simulink library "lib_Hand"  (R2022b)
settings: Solver=VariableStepAuto  StartTime=0.0  StopTime=10.0  RelTol=1e-3
settings Model: Creator=li_ju  LastModifiedBy=ge26jow

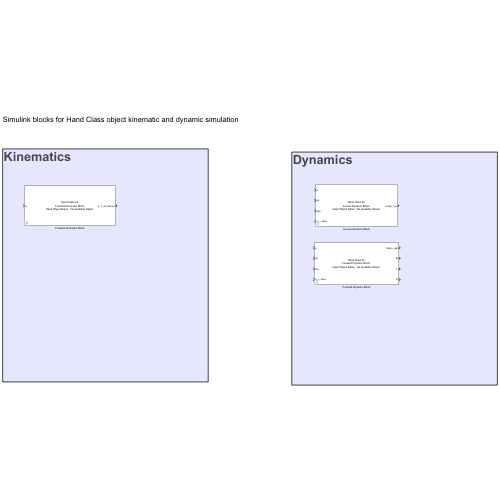
[thumbnail: Simulink's stored preview of the top-level diagram]
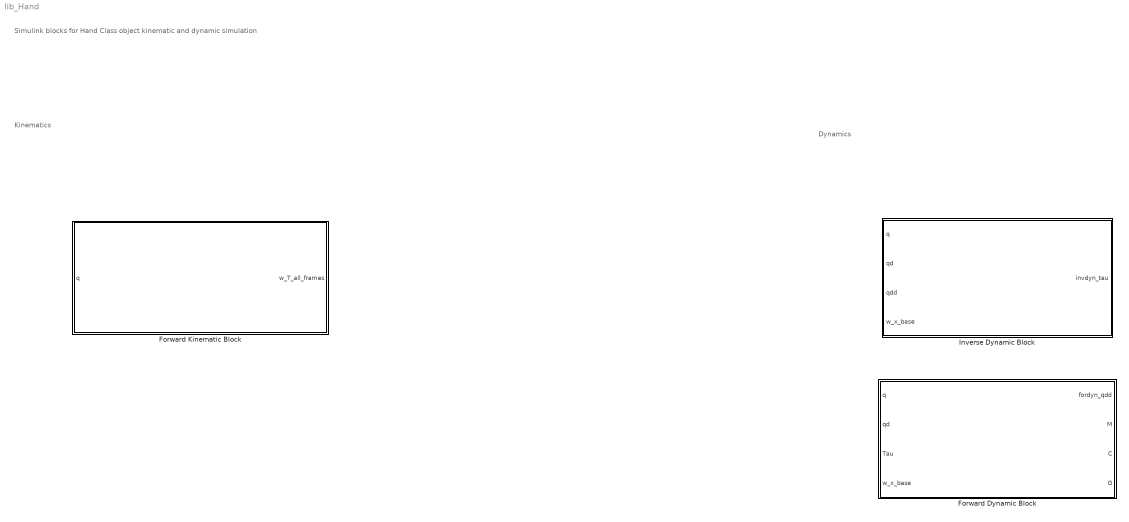
== system lib_Hand ==
  note: Kinematics
  note: Simulink blocks for Hand Class object kinematic and dynamic simulation
  note: Dynamics
  Forward Dynamic Block : Subsystem  mask{hand=0}
      mask prompts: hand "Hand Model Object"
      mask init:
      | if isa(hand,"Hand")
      |        handname = hand.name;
      |    else
      |         handname = 'No Available Object';
      |    end
      mask Display:
      | fprintf(['Hand Class lib \n' ...
      |     'Forward Dynamic Block \n' ...
      |     'Hand Object Name:  %s '], handname)
  Forward Kinematic Block : Subsystem  mask{hand=0}
      mask prompts: hand "Hand Model Object"
      mask init:
      | if isa(hand,"Hand")
      |        handname = hand.name;
      |    else
      |         handname = 'No Available Object';
      |    end
      mask Display:
      | fprintf(['Hand Class lib \n' ...
      |     'Forward Kinematic Block \n' ...
      |     'Hand Object Name:  %s '], handname)
  Inverse Dynamic Block : Subsystem  mask{hand=0}
      mask prompts: hand "Hand Model Object"
      mask init:
      | if isa(hand,"Hand")
      |        handname = hand.name;
      |    else
      |         handname = 'No Available Object';
      |    end
      mask Display:
      | fprintf(['Hand Class lib \n' ...
      |     'Inverse Dynamic Block \n' ...
      |     'Hand Object Name:  %s '], handname)

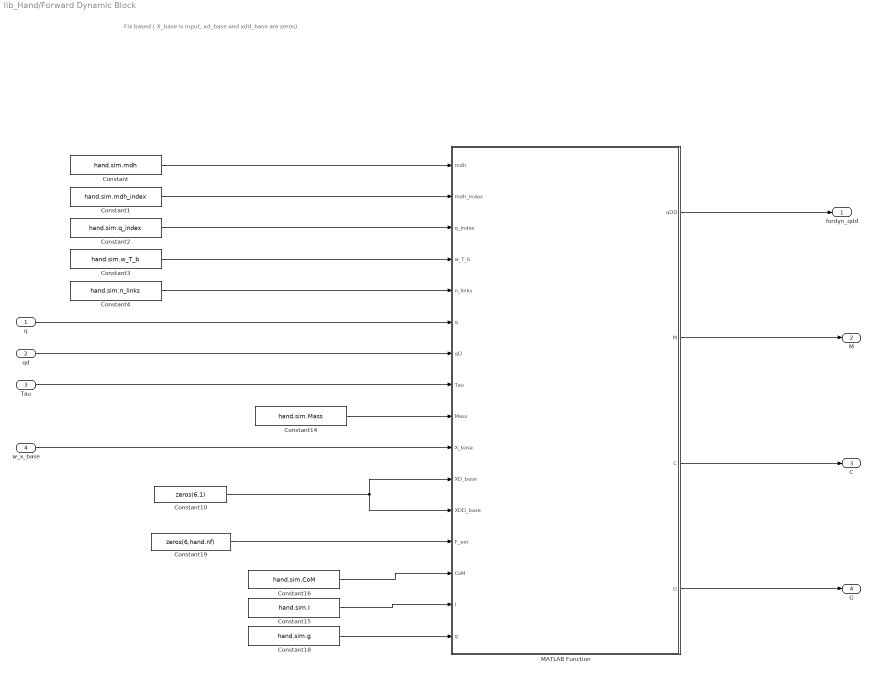
== system lib_Hand/Forward Dynamic Block ==
  note: Fix based ( X_base is input, xd_base and xdd_base are zeros)
  q : Inport
  qd : Inport  Port=2
  Tau : Inport  Port=3
  w_x_base : Inport  Port=4
  Constant : Constant  Value=hand.sim.mdh
  Constant1 : Constant  Value=hand.sim.mdh_index
  Constant10 : Constant  Value=zeros(6,1)  VectorParams1D=off
  Constant14 : Constant  Value=hand.sim.Mass  VectorParams1D=off
  Constant15 : Constant  Value=hand.sim.I
  Constant16 : Constant  Value=hand.sim.CoM
  Constant18 : Constant  Value=hand.sim.g  VectorParams1D=off
  Constant19 : Constant  Value=zeros(6,hand.nf)
  Constant2 : Constant  Value=hand.sim.q_index
  Constant3 : Constant  Value=hand.sim.w_T_b
  Constant4 : Constant  Value=hand.sim.n_links  VectorParams1D=off
  MATLAB Function : MATLAB Function  TreatAsAtomicUnit=on
  fordyn_qdd : Outport
  M : Outport  Port=2
  C : Outport  Port=3
  G : Outport  Port=4
  wires:
  Constant14/1 -> MATLAB Function/9(Mass)
  MATLAB Function/1(qDD) -> fordyn_qdd/1
  Constant10/1 -> MATLAB Function/12(XDD_base), MATLAB Function/11(XD_base)
  Constant15/1 -> MATLAB Function/15(I)
  Constant19/1 -> MATLAB Function/13(F_ext)
  Constant16/1 -> MATLAB Function/14(CoM)
  qd/1 -> MATLAB Function/7(qD)
  Constant2/1 -> MATLAB Function/3(q_index)
  q/1 -> MATLAB Function/6(q)
  Constant/1 -> MATLAB Function/1(mdh)
  Constant3/1 -> MATLAB Function/4(w_T_b)
  Constant1/1 -> MATLAB Function/2(mdh_index)
  Constant18/1 -> MATLAB Function/16(g)
  Constant4/1 -> MATLAB Function/5(n_links)
  Tau/1 -> MATLAB Function/8(Tau)
  w_x_base/1 -> MATLAB Function/10(X_base)
  MATLAB Function/2(M) -> M/1
  MATLAB Function/3(C) -> C/1
  MATLAB Function/4(G) -> G/1

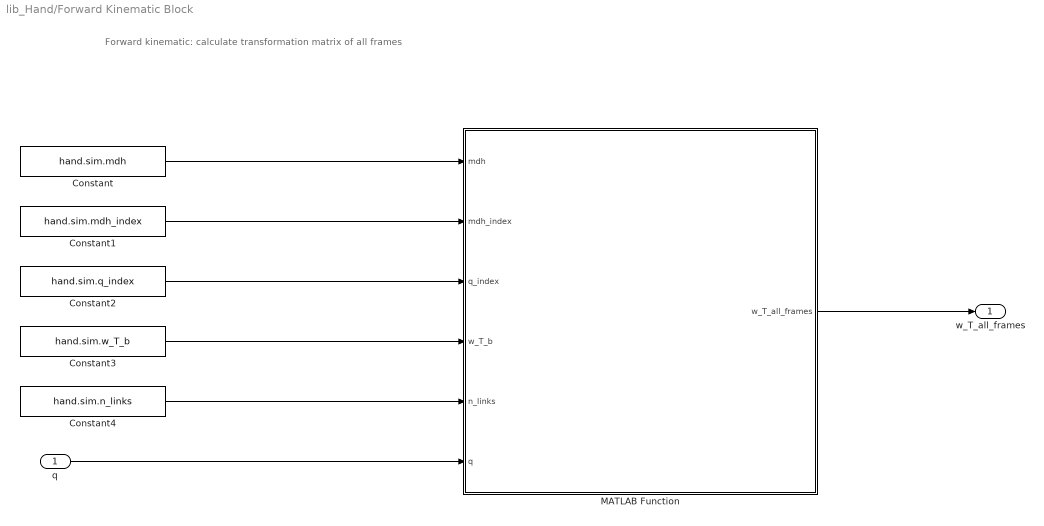
== system lib_Hand/Forward Kinematic Block ==
  note: Forward kinematic: calculate transformation matrix of all frames
  q : Inport
  Constant : Constant  Value=hand.sim.mdh
  Constant1 : Constant  Value=hand.sim.mdh_index
  Constant2 : Constant  Value=hand.sim.q_index
  Constant3 : Constant  Value=hand.sim.w_T_b
  Constant4 : Constant  Value=hand.sim.n_links  VectorParams1D=off
  MATLAB Function : MATLAB Function  TreatAsAtomicUnit=on
  w_T_all_frames : Outport
  wires:
  MATLAB Function/1(w_T_all_frames) -> w_T_all_frames/1
  Constant2/1 -> MATLAB Function/3(q_index)
  q/1 -> MATLAB Function/6(q)
  Constant/1 -> MATLAB Function/1(mdh)
  Constant3/1 -> MATLAB Function/4(w_T_b)
  Constant1/1 -> MATLAB Function/2(mdh_index)
  Constant4/1 -> MATLAB Function/5(n_links)

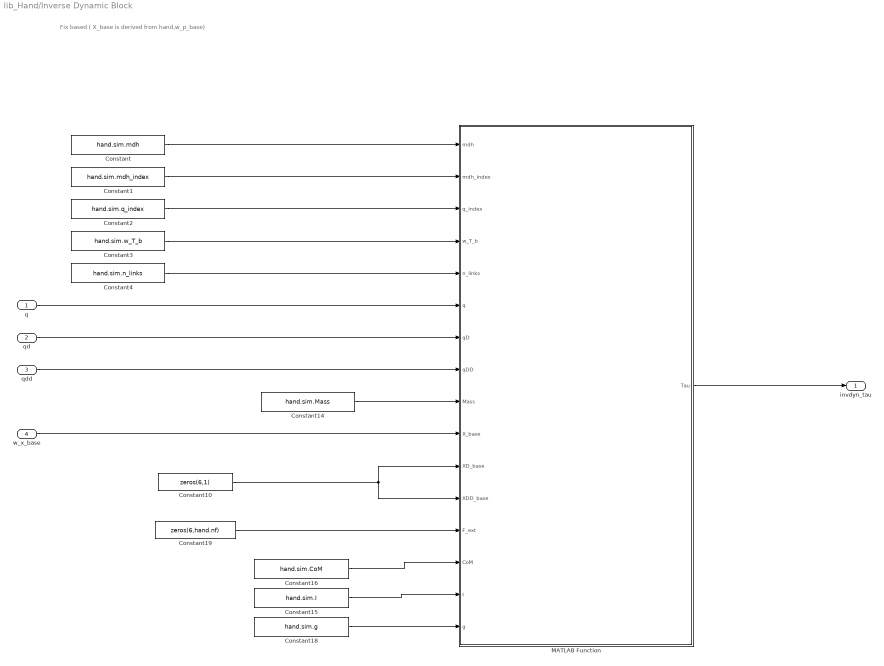
== system lib_Hand/Inverse Dynamic Block ==
  note: Fix based ( X_base is derived from hand,w_p_base)
  q : Inport
  qd : Inport  Port=2
  qdd : Inport  Port=3
  w_x_base : Inport  Port=4
  Constant : Constant  Value=hand.sim.mdh
  Constant1 : Constant  Value=hand.sim.mdh_index
  Constant10 : Constant  Value=zeros(6,1)  VectorParams1D=off
  Constant14 : Constant  Value=hand.sim.Mass  VectorParams1D=off
  Constant15 : Constant  Value=hand.sim.I
  Constant16 : Constant  Value=hand.sim.CoM
  Constant18 : Constant  Value=hand.sim.g  VectorParams1D=off
  Constant19 : Constant  Value=zeros(6,hand.nf)
  Constant2 : Constant  Value=hand.sim.q_index
  Constant3 : Constant  Value=hand.sim.w_T_b
  Constant4 : Constant  Value=hand.sim.n_links  VectorParams1D=off
  MATLAB Function : MATLAB Function  TreatAsAtomicUnit=on
  invdyn_tau : Outport
  wires:
  Constant14/1 -> MATLAB Function/9(Mass)
  MATLAB Function/1(Tau) -> invdyn_tau/1
  Constant10/1 -> MATLAB Function/11(XD_base), MATLAB Function/12(XDD_base)
  Constant15/1 -> MATLAB Function/15(I)
  Constant19/1 -> MATLAB Function/13(F_ext)
  Constant16/1 -> MATLAB Function/14(CoM)
  qd/1 -> MATLAB Function/7(qD)
  Constant2/1 -> MATLAB Function/3(q_index)
  q/1 -> MATLAB Function/6(q)
  Constant/1 -> MATLAB Function/1(mdh)
  Constant3/1 -> MATLAB Function/4(w_T_b)
  Constant1/1 -> MATLAB Function/2(mdh_index)
  Constant18/1 -> MATLAB Function/16(g)
  Constant4/1 -> MATLAB Function/5(n_links)
  qdd/1 -> MATLAB Function/8(qDD)
  w_x_base/1 -> MATLAB Function/10(X_base)

== matlab function lib_Hand/Forward Kinematic Block/MATLAB Function ==
  data: w_T_all_frames output; mdh input; mdh_index input; q_index input; w_T_b input; n_links input; q input
function w_T_all_frames = fcn(mdh, mdh_index, q_index, w_T_b, n_links, q)

% calculate transformation matrix of frames
w_T_all_frames = sim_w_T_all_frames_from_q(mdh,mdh_index,q_index,w_T_b,n_links,q);

== matlab function lib_Hand/Inverse Dynamic Block/MATLAB Function ==
  data: Tau output; mdh input; mdh_index input; q_index input; w_T_b input; n_links input; q input; qD input; qDD input; Mass input; X_base input; XD_base input; XDD_base input; F_ext input; CoM input; I input; g input
function Tau = fcn(mdh, mdh_index, q_index, w_T_b, n_links, q, qD, qDD, Mass, X_base, XD_base,XDD_base, F_ext, CoM, I, g)

% calculate transformation matrix of frames
w_T_all_frames = sim_w_T_all_frames_from_q(mdh,mdh_index,q_index,w_T_b,n_links,q);
% calculate inverse dynamics
Tau = invdyn_ne_T(w_T_all_frames,qD,qDD, n_links, q_index, Mass, X_base, XD_base,XDD_base, F_ext, CoM, I, g);

== matlab function lib_Hand/Forward Dynamic Block/MATLAB Function ==
  data: qDD output; mdh input; mdh_index input; q_index input; w_T_b input; n_links input; q input; qD input; Tau input; Mass input; X_base input; XD_base input; XDD_base input; F_ext input; CoM input; I input; g input; M output; C output; G output
function [qDD,M,C,G] = fcn(mdh, mdh_index, q_index, w_T_b, n_links, q, qD, Tau, Mass, X_base, XD_base,XDD_base, F_ext, CoM, I, g)

% calculate transformation matrix of frames
w_T_all_frames = sim_w_T_all_frames_from_q(mdh,mdh_index,q_index,w_T_b,n_links,q);
% calculate forward dynamics
[qDD,M,C,G] = fordyn_ne_T(w_T_all_frames,qD,Tau, n_links, q_index, Mass, X_base, XD_base,XDD_base, F_ext, CoM, I, g);
